simulink model "Dianlan_low_residence"  (R2021a)
settings: Solver=VariableStepAuto  StartTime=0.0  StopTime=20e-6  RelTol=1e-3
libraries: spsGroundLib x4, spsSeriesRLCBranchLib x3, spsVoltageMeasurementLib x3, spsDistributedParametersLineLib x2, spsControlledVoltageSourceLib x1, spspowerguiLib x1
settings Model: Creator=张瑞  LastModifiedBy=张瑞

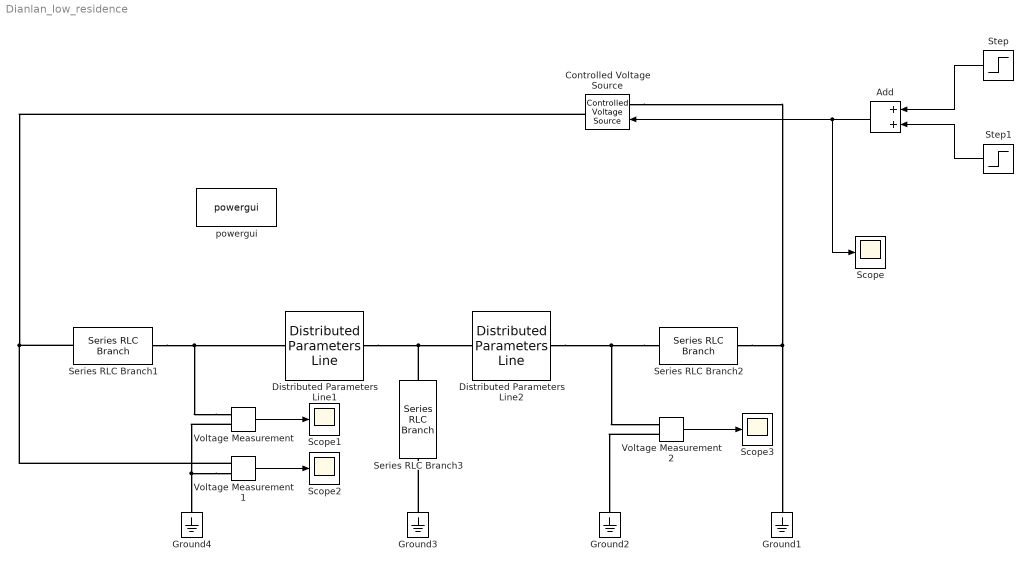
== system Dianlan_low_residence ==
  Add : Sum
  Controlled Voltage Source : spsControlledVoltageSourceLib/Controlled Voltage Source  Initialize=off  Source_Type=AC  Amplitude=0  Phase=0  Frequency=0  Measurements=Voltage
  Distributed Parameters Line1 : spsDistributedParametersLineLib/Distributed Parameters Line  Phases=1  Length=0.01  Frequency=1000  Resistance=1.8E-1  Inductance=2.75E-4  Capacitance=5.57E-7  x1=[-1.3e-07 0;-1.2e-07 0;-1.1e-07 0;-1e-07 0;-9e-08 0;-8e-08 0;-7e-08 0;-6e-08 0;-5e-08 0;-4e-08 0;-3e-08 0;-2e-08 0;-1e-08 0]  x2=[-1.3e-07 0;-1.2e-07 0;-1.1e-07 0;-1e-07 0;-9e-08 0;-8e-08 0;-7e-08 0;-6e-08 0;-5e-08 0;-4e-08 0;-3e-08 0;-2e-08 0;-1e-08 0]  x3=[-1.3e-07 0;-1.2e-07 0;-1.1e-07 0;-1e-07 0;-9e-08 0;-8e-08 0;-7e-08 0;-6e-08 0;-5e-08 0;-4e-08 0;-3e-08 0;-2e-08 0;-1e-08 0]  x4=[-1.3e-07 0;-1.2e-07 0;-1.1e-07 0;-1e-07 0;-9e-08 0;-8e-08 0;-7e-08 0;-6e-08 0;-5e-08 0;-4e-08 0;-3e-08 0;-2e-08 0;-1e-08 0]  x5=1.23763888109577e-07  V1=ones(3,3)  V2=ones(3,3)  I1=ones(3,3)  I2=ones(3,3)  nHarmo=1  Measurements=Phase-to-ground voltages  Decoupling=off  VsMag0=0  VrMag0=0  VsAngle0=0  VrAngle0=0  IsMag0=0  IrMag0=0  IsAngle0=0  IrAngle0=0
      settings: SourceProductBaseCode=PS
  Distributed Parameters Line2 : spsDistributedParametersLineLib/Distributed Parameters Line  Phases=1  Length=1.99  Frequency=1000  Resistance=1.8E-1  Inductance=2.75E-4  Capacitance=5.57E-7  x1=[-2.463e-05 0;-2.462e-05 0;-2.461e-05 0;-2.46e-05 0;-2.459e-05 0;-2.458e-05 0;-2.457e-05 0;-2.456e-05 0;-2.455e-05 0;-2.454e-05 0;-2.453e-05 0;-2.452e-05 0;-2.451e-05 0;-2.45e-05 0;-2.449e-05 0;-2.448e-05 0;-2.447e-05 0;-2.446e-05 0;-2.445e-05 0;-2.444e-05 0;-2.443e-05 0;-2.442e-05 0;-2.441e-05 0;-2.44e-05 0;-2.439e-05 0;-2.438e-05 0;-2.437e-05 0;-2.436e-05 0;-2.435e-05 0;-2.434e-05 0;-2.433e-05 0;-2.432e-05 0;-2.431e-05 0;-2.43e-05 0;-2.429e-05 0;-2.428e-05 0;-2.427e-05 0;-2.426e-05 0;-2.425e-05 0;-2.424e-05 0;-2.423e-05 0;-2.422e-05 0;-2.421e-05 0;-2.42e-05 0;-2.419e-05 0;-2.418e-05 0;-2.417e-05 0;-2.416e-05 0;-2.415e-05 0;-2.414e-05 0;-2.413e-05 0;-2.412e-05 0;-2.411e-05 0;-2.41e-05 0;-2.409e-05 0;-2.408e-05 0;-2.407e-05 0;-2.406e-05 0;-2.405e-05 0;-2.404e-05 0;-2.403e-05 0;-2.402e-05 0;-2.401e-05 0;-2.4e-05 0;-2.399e-05 0;-2.398e-05 0;-2.397e-05 0;-2.396e-05 0;-2.395e-05 0;-2.394e-05 0;-2.393e-05 0;-2.392e-05 0;-2.391e-05 0;-2.39e-05 0;-2.389e-05 0;-2.388e-05 0;-2.387e-05 0;-2.386e-05 0;-2.385e-05 0;-2.384e-05 0;-2.383e-05 0;-2.382e-05 0;-2.381e-05 0;-2.38e-05 0;-2.379e-05 0;-2.378e-05 0;-2.377e-05 0;-2.376e-05 0;-2.375e-05 0;-2.374e-05 0;-2.373e-05 0;-2.372e-05 0;-2.371e-05 0;-2.37e-05 0;-2.369e-05 0;-2.368e-05 0;-2.367e-05 0;-2.366e-05 0;-2.365e-05 0;-2.364e-05 0;-2.363e-05 0;-2.362e-05 0;-2.361e-05 0;-2.36e-05 0;-2.359e-05 0;-2.358e-05 0;-2.357e-05 0;-2.356e-05 0;-2.355e-05 0;-2.354e-05 0;-2.353e-05 0;-2.352e-05 0;-2.351e-05 0;-2.35e-05 0;-2.349e-05 0;-2.348e-05 0;-2.347e-05 0;-2.346e-05 0;-2.345e-05 0;-2.344e-05 0;-2.343e-05 0;-2.342e-05 0;-2.341e-05 0;-2.34e-05 0;-2.339e-05 0;-2.338e-05 0;-2.337e-05 0;-2.336e-05 0;-2.335e-05 0;-2.334e-05 0;-2.333e-05 0;-2.332e-05 0;-2.331e-05 0;-2.33e-05 0;-2.329e-05 0;-2.328e-05 0;-2.327e-05 0;-2.326e-05 0;-2.325e-05 0;-2.324e-05 0;-2.323e-05 0;-2.322e-05 0;-2.321e-05 0;-2.32e-05 0;-2.319e-05 0;-2.318e-05 0;-2.317e-05 0;-2.316e-05 0;-2.315e-05 0;-2.314e-05 0;-2.313e-05 0;-2.312e-05 0;-2.311e-05 0;-2.31e-05 0;-2.309e-05 0;-2.308e-05 0;-2.307e-05 0;-2.306e-05 0;-2.305e-05 0;-2.304e-05 0;-2.303e-05 0;-2.302e-05 0;-2.301e-05 0;-2.3e-05 0;-2.299e-05 0;-2.298e-05 0;-2.297e-05 0;-2.296e-05 0;-2.295e-05 0;-2.294e-05 0;-2.293e-05 0;-2.292e-05 0;-2.291e-05 0;-2.29e-05 0;-2.289e-05 0;-2.288e-05 0;-2.287e-05 0;-2.286e-05 0;-2.285e-05 0;-2.284e-05 0;-2.283e-05 0;-2.282e-05 0;-2.281e-05 0;-2.28e-05 0;-2.279e-05 0;-2.278e-05 0;-2.277e-05 0;-2.276e-05 0;-2.275e-05 0;-2.274e-05 0;-2.273e-05 0;-2.272e-05 0;-2.271e-05 0;-2.27e-05 0;-2.269e-05 0;-2.268e-05 0;-2.267e-05 0;-2.266e-05 0;-2.265e-05 0;-2.264e-05 0;-2.263e-05 0;-2.262e-05 0;-2.261e-05 0;-2.26e-05 0;-2.259e-05 0;-2.258e-05 0;-2.257e-05 0;-2.256e-05 0;-2.255e-05 0;-2.254e-05 0;-2.253e-05 0;-2.252e-05 0;-2.251e-05 0;-2.25e-05 0;-2.249e-05 0;-2.248e-05 0;-2.247e-05 0;-2.246e-05 0;-2.245e-05 0;-2.244e-05 0;-2.243e-05 0;-2.242e-05 0;-2.241e-05 0;-2.24e-05 0;-2.239e-05 0;-2.238e-05 0;-2.237e-05 0;-2.236e-05 0;-2.235e-05 0;-2.234e-05 0;-2.233e-05 0;-2.232e-05 0;-2.231e-05 0;-2.23e-05 0;-2.229e-05 0;-2.228e-05 0;-2.227e-05 0;-2.226e-05 0;-2.225e-05 0;-2.224e-05 0;-2.223e-05 0;-2.222e-05 0;-2.221e-05 0;-2.22e-05 0;-2.219e-05 0;-2.218e-05 0;-2.217e-05 0;-2.216e-05 0;-2.215e-05 0;-2.214e-05 0;-2.213e-05 0;-2.212e-05 0;-2.211e-05 0;-2.21e-05 0;-2.209e-05 0;-2.208e-05 0;-2.207e-05 0;-2.206e-05 0;-2.205e-05 0;-2.204e-05 0;-2.203e-05 0;-2.202e-05 0;-2.201e-05 0;-2.2e-05 0;-2.199e-05 0;-2.198e-05 0;-2.197e-05 0;-2.196e-05 0;-2.195e-05 0;-2.194e-05 0;-2.193e-05 0;-2.192e-05 0;-2.191e-05 0;-2.19e-05 0;-2.189e-05 0;-2.188e-05 0;-2.187e-05 0;-2.186e-05 0;-2.185e-05 0;-2.184e-05 0;-2.183e-05 0;-2.182e-05 0;-2.181e-05 0;-2.18e-05 0;-2.179e-05 0;-2.178e-05 0;-2.177e-05 0;-2.176e-05 0;-2.175e-05 0;-2.174e-05 0;-2.173e-05 0;-2.172e-05 0;-2.171e-05 0;-2.17e-05 0;-2.169e-05 0;-2.168e-05 0;-2.167e-05 0;-2.166e-05 0;-2.165e-05 0;-2.164e-05 0;-2.163e-05 0;-2.162e-05 0;-2.161e-05 0;-2.16e-05 0;-2.159e-05 0;-2.158e-05 0;-2.157e-05 0;-2.156e-05 0;-2.155e-05 0;-2.154e-05 0 ...(+26615 chars)]  x2=[-2.463e-05 0;-2.462e-05 0;-2.461e-05 0;-2.46e-05 0;-2.459e-05 0;-2.458e-05 0;-2.457e-05 0;-2.456e-05 0;-2.455e-05 0;-2.454e-05 0;-2.453e-05 0;-2.452e-05 0;-2.451e-05 0;-2.45e-05 0;-2.449e-05 0;-2.448e-05 0;-2.447e-05 0;-2.446e-05 0;-2.445e-05 0;-2.444e-05 0;-2.443e-05 0;-2.442e-05 0;-2.441e-05 0;-2.44e-05 0;-2.439e-05 0;-2.438e-05 0;-2.437e-05 0;-2.436e-05 0;-2.435e-05 0;-2.434e-05 0;-2.433e-05 0;-2.432e-05 0;-2.431e-05 0;-2.43e-05 0;-2.429e-05 0;-2.428e-05 0;-2.427e-05 0;-2.426e-05 0;-2.425e-05 0;-2.424e-05 0;-2.423e-05 0;-2.422e-05 0;-2.421e-05 0;-2.42e-05 0;-2.419e-05 0;-2.418e-05 0;-2.417e-05 0;-2.416e-05 0;-2.415e-05 0;-2.414e-05 0;-2.413e-05 0;-2.412e-05 0;-2.411e-05 0;-2.41e-05 0;-2.409e-05 0;-2.408e-05 0;-2.407e-05 0;-2.406e-05 0;-2.405e-05 0;-2.404e-05 0;-2.403e-05 0;-2.402e-05 0;-2.401e-05 0;-2.4e-05 0;-2.399e-05 0;-2.398e-05 0;-2.397e-05 0;-2.396e-05 0;-2.395e-05 0;-2.394e-05 0;-2.393e-05 0;-2.392e-05 0;-2.391e-05 0;-2.39e-05 0;-2.389e-05 0;-2.388e-05 0;-2.387e-05 0;-2.386e-05 0;-2.385e-05 0;-2.384e-05 0;-2.383e-05 0;-2.382e-05 0;-2.381e-05 0;-2.38e-05 0;-2.379e-05 0;-2.378e-05 0;-2.377e-05 0;-2.376e-05 0;-2.375e-05 0;-2.374e-05 0;-2.373e-05 0;-2.372e-05 0;-2.371e-05 0;-2.37e-05 0;-2.369e-05 0;-2.368e-05 0;-2.367e-05 0;-2.366e-05 0;-2.365e-05 0;-2.364e-05 0;-2.363e-05 0;-2.362e-05 0;-2.361e-05 0;-2.36e-05 0;-2.359e-05 0;-2.358e-05 0;-2.357e-05 0;-2.356e-05 0;-2.355e-05 0;-2.354e-05 0;-2.353e-05 0;-2.352e-05 0;-2.351e-05 0;-2.35e-05 0;-2.349e-05 0;-2.348e-05 0;-2.347e-05 0;-2.346e-05 0;-2.345e-05 0;-2.344e-05 0;-2.343e-05 0;-2.342e-05 0;-2.341e-05 0;-2.34e-05 0;-2.339e-05 0;-2.338e-05 0;-2.337e-05 0;-2.336e-05 0;-2.335e-05 0;-2.334e-05 0;-2.333e-05 0;-2.332e-05 0;-2.331e-05 0;-2.33e-05 0;-2.329e-05 0;-2.328e-05 0;-2.327e-05 0;-2.326e-05 0;-2.325e-05 0;-2.324e-05 0;-2.323e-05 0;-2.322e-05 0;-2.321e-05 0;-2.32e-05 0;-2.319e-05 0;-2.318e-05 0;-2.317e-05 0;-2.316e-05 0;-2.315e-05 0;-2.314e-05 0;-2.313e-05 0;-2.312e-05 0;-2.311e-05 0;-2.31e-05 0;-2.309e-05 0;-2.308e-05 0;-2.307e-05 0;-2.306e-05 0;-2.305e-05 0;-2.304e-05 0;-2.303e-05 0;-2.302e-05 0;-2.301e-05 0;-2.3e-05 0;-2.299e-05 0;-2.298e-05 0;-2.297e-05 0;-2.296e-05 0;-2.295e-05 0;-2.294e-05 0;-2.293e-05 0;-2.292e-05 0;-2.291e-05 0;-2.29e-05 0;-2.289e-05 0;-2.288e-05 0;-2.287e-05 0;-2.286e-05 0;-2.285e-05 0;-2.284e-05 0;-2.283e-05 0;-2.282e-05 0;-2.281e-05 0;-2.28e-05 0;-2.279e-05 0;-2.278e-05 0;-2.277e-05 0;-2.276e-05 0;-2.275e-05 0;-2.274e-05 0;-2.273e-05 0;-2.272e-05 0;-2.271e-05 0;-2.27e-05 0;-2.269e-05 0;-2.268e-05 0;-2.267e-05 0;-2.266e-05 0;-2.265e-05 0;-2.264e-05 0;-2.263e-05 0;-2.262e-05 0;-2.261e-05 0;-2.26e-05 0;-2.259e-05 0;-2.258e-05 0;-2.257e-05 0;-2.256e-05 0;-2.255e-05 0;-2.254e-05 0;-2.253e-05 0;-2.252e-05 0;-2.251e-05 0;-2.25e-05 0;-2.249e-05 0;-2.248e-05 0;-2.247e-05 0;-2.246e-05 0;-2.245e-05 0;-2.244e-05 0;-2.243e-05 0;-2.242e-05 0;-2.241e-05 0;-2.24e-05 0;-2.239e-05 0;-2.238e-05 0;-2.237e-05 0;-2.236e-05 0;-2.235e-05 0;-2.234e-05 0;-2.233e-05 0;-2.232e-05 0;-2.231e-05 0;-2.23e-05 0;-2.229e-05 0;-2.228e-05 0;-2.227e-05 0;-2.226e-05 0;-2.225e-05 0;-2.224e-05 0;-2.223e-05 0;-2.222e-05 0;-2.221e-05 0;-2.22e-05 0;-2.219e-05 0;-2.218e-05 0;-2.217e-05 0;-2.216e-05 0;-2.215e-05 0;-2.214e-05 0;-2.213e-05 0;-2.212e-05 0;-2.211e-05 0;-2.21e-05 0;-2.209e-05 0;-2.208e-05 0;-2.207e-05 0;-2.206e-05 0;-2.205e-05 0;-2.204e-05 0;-2.203e-05 0;-2.202e-05 0;-2.201e-05 0;-2.2e-05 0;-2.199e-05 0;-2.198e-05 0;-2.197e-05 0;-2.196e-05 0;-2.195e-05 0;-2.194e-05 0;-2.193e-05 0;-2.192e-05 0;-2.191e-05 0;-2.19e-05 0;-2.189e-05 0;-2.188e-05 0;-2.187e-05 0;-2.186e-05 0;-2.185e-05 0;-2.184e-05 0;-2.183e-05 0;-2.182e-05 0;-2.181e-05 0;-2.18e-05 0;-2.179e-05 0;-2.178e-05 0;-2.177e-05 0;-2.176e-05 0;-2.175e-05 0;-2.174e-05 0;-2.173e-05 0;-2.172e-05 0;-2.171e-05 0;-2.17e-05 0;-2.169e-05 0;-2.168e-05 0;-2.167e-05 0;-2.166e-05 0;-2.165e-05 0;-2.164e-05 0;-2.163e-05 0;-2.162e-05 0;-2.161e-05 0;-2.16e-05 0;-2.159e-05 0;-2.158e-05 0;-2.157e-05 0;-2.156e-05 0;-2.155e-05 0;-2.154e-05 0 ...(+26615 chars)]  x3=[-2.463e-05 0;-2.462e-05 0;-2.461e-05 0;-2.46e-05 0;-2.459e-05 0;-2.458e-05 0;-2.457e-05 0;-2.456e-05 0;-2.455e-05 0;-2.454e-05 0;-2.453e-05 0;-2.452e-05 0;-2.451e-05 0;-2.45e-05 0;-2.449e-05 0;-2.448e-05 0;-2.447e-05 0;-2.446e-05 0;-2.445e-05 0;-2.444e-05 0;-2.443e-05 0;-2.442e-05 0;-2.441e-05 0;-2.44e-05 0;-2.439e-05 0;-2.438e-05 0;-2.437e-05 0;-2.436e-05 0;-2.435e-05 0;-2.434e-05 0;-2.433e-05 0;-2.432e-05 0;-2.431e-05 0;-2.43e-05 0;-2.429e-05 0;-2.428e-05 0;-2.427e-05 0;-2.426e-05 0;-2.425e-05 0;-2.424e-05 0;-2.423e-05 0;-2.422e-05 0;-2.421e-05 0;-2.42e-05 0;-2.419e-05 0;-2.418e-05 0;-2.417e-05 0;-2.416e-05 0;-2.415e-05 0;-2.414e-05 0;-2.413e-05 0;-2.412e-05 0;-2.411e-05 0;-2.41e-05 0;-2.409e-05 0;-2.408e-05 0;-2.407e-05 0;-2.406e-05 0;-2.405e-05 0;-2.404e-05 0;-2.403e-05 0;-2.402e-05 0;-2.401e-05 0;-2.4e-05 0;-2.399e-05 0;-2.398e-05 0;-2.397e-05 0;-2.396e-05 0;-2.395e-05 0;-2.394e-05 0;-2.393e-05 0;-2.392e-05 0;-2.391e-05 0;-2.39e-05 0;-2.389e-05 0;-2.388e-05 0;-2.387e-05 0;-2.386e-05 0;-2.385e-05 0;-2.384e-05 0;-2.383e-05 0;-2.382e-05 0;-2.381e-05 0;-2.38e-05 0;-2.379e-05 0;-2.378e-05 0;-2.377e-05 0;-2.376e-05 0;-2.375e-05 0;-2.374e-05 0;-2.373e-05 0;-2.372e-05 0;-2.371e-05 0;-2.37e-05 0;-2.369e-05 0;-2.368e-05 0;-2.367e-05 0;-2.366e-05 0;-2.365e-05 0;-2.364e-05 0;-2.363e-05 0;-2.362e-05 0;-2.361e-05 0;-2.36e-05 0;-2.359e-05 0;-2.358e-05 0;-2.357e-05 0;-2.356e-05 0;-2.355e-05 0;-2.354e-05 0;-2.353e-05 0;-2.352e-05 0;-2.351e-05 0;-2.35e-05 0;-2.349e-05 0;-2.348e-05 0;-2.347e-05 0;-2.346e-05 0;-2.345e-05 0;-2.344e-05 0;-2.343e-05 0;-2.342e-05 0;-2.341e-05 0;-2.34e-05 0;-2.339e-05 0;-2.338e-05 0;-2.337e-05 0;-2.336e-05 0;-2.335e-05 0;-2.334e-05 0;-2.333e-05 0;-2.332e-05 0;-2.331e-05 0;-2.33e-05 0;-2.329e-05 0;-2.328e-05 0;-2.327e-05 0;-2.326e-05 0;-2.325e-05 0;-2.324e-05 0;-2.323e-05 0;-2.322e-05 0;-2.321e-05 0;-2.32e-05 0;-2.319e-05 0;-2.318e-05 0;-2.317e-05 0;-2.316e-05 0;-2.315e-05 0;-2.314e-05 0;-2.313e-05 0;-2.312e-05 0;-2.311e-05 0;-2.31e-05 0;-2.309e-05 0;-2.308e-05 0;-2.307e-05 0;-2.306e-05 0;-2.305e-05 0;-2.304e-05 0;-2.303e-05 0;-2.302e-05 0;-2.301e-05 0;-2.3e-05 0;-2.299e-05 0;-2.298e-05 0;-2.297e-05 0;-2.296e-05 0;-2.295e-05 0;-2.294e-05 0;-2.293e-05 0;-2.292e-05 0;-2.291e-05 0;-2.29e-05 0;-2.289e-05 0;-2.288e-05 0;-2.287e-05 0;-2.286e-05 0;-2.285e-05 0;-2.284e-05 0;-2.283e-05 0;-2.282e-05 0;-2.281e-05 0;-2.28e-05 0;-2.279e-05 0;-2.278e-05 0;-2.277e-05 0;-2.276e-05 0;-2.275e-05 0;-2.274e-05 0;-2.273e-05 0;-2.272e-05 0;-2.271e-05 0;-2.27e-05 0;-2.269e-05 0;-2.268e-05 0;-2.267e-05 0;-2.266e-05 0;-2.265e-05 0;-2.264e-05 0;-2.263e-05 0;-2.262e-05 0;-2.261e-05 0;-2.26e-05 0;-2.259e-05 0;-2.258e-05 0;-2.257e-05 0;-2.256e-05 0;-2.255e-05 0;-2.254e-05 0;-2.253e-05 0;-2.252e-05 0;-2.251e-05 0;-2.25e-05 0;-2.249e-05 0;-2.248e-05 0;-2.247e-05 0;-2.246e-05 0;-2.245e-05 0;-2.244e-05 0;-2.243e-05 0;-2.242e-05 0;-2.241e-05 0;-2.24e-05 0;-2.239e-05 0;-2.238e-05 0;-2.237e-05 0;-2.236e-05 0;-2.235e-05 0;-2.234e-05 0;-2.233e-05 0;-2.232e-05 0;-2.231e-05 0;-2.23e-05 0;-2.229e-05 0;-2.228e-05 0;-2.227e-05 0;-2.226e-05 0;-2.225e-05 0;-2.224e-05 0;-2.223e-05 0;-2.222e-05 0;-2.221e-05 0;-2.22e-05 0;-2.219e-05 0;-2.218e-05 0;-2.217e-05 0;-2.216e-05 0;-2.215e-05 0;-2.214e-05 0;-2.213e-05 0;-2.212e-05 0;-2.211e-05 0;-2.21e-05 0;-2.209e-05 0;-2.208e-05 0;-2.207e-05 0;-2.206e-05 0;-2.205e-05 0;-2.204e-05 0;-2.203e-05 0;-2.202e-05 0;-2.201e-05 0;-2.2e-05 0;-2.199e-05 0;-2.198e-05 0;-2.197e-05 0;-2.196e-05 0;-2.195e-05 0;-2.194e-05 0;-2.193e-05 0;-2.192e-05 0;-2.191e-05 0;-2.19e-05 0;-2.189e-05 0;-2.188e-05 0;-2.187e-05 0;-2.186e-05 0;-2.185e-05 0;-2.184e-05 0;-2.183e-05 0;-2.182e-05 0;-2.181e-05 0;-2.18e-05 0;-2.179e-05 0;-2.178e-05 0;-2.177e-05 0;-2.176e-05 0;-2.175e-05 0;-2.174e-05 0;-2.173e-05 0;-2.172e-05 0;-2.171e-05 0;-2.17e-05 0;-2.169e-05 0;-2.168e-05 0;-2.167e-05 0;-2.166e-05 0;-2.165e-05 0;-2.164e-05 0;-2.163e-05 0;-2.162e-05 0;-2.161e-05 0;-2.16e-05 0;-2.159e-05 0;-2.158e-05 0;-2.157e-05 0;-2.156e-05 0;-2.155e-05 0;-2.154e-05 0 ...(+26615 chars)]  x4=[-2.463e-05 0;-2.462e-05 0;-2.461e-05 0;-2.46e-05 0;-2.459e-05 0;-2.458e-05 0;-2.457e-05 0;-2.456e-05 0;-2.455e-05 0;-2.454e-05 0;-2.453e-05 0;-2.452e-05 0;-2.451e-05 0;-2.45e-05 0;-2.449e-05 0;-2.448e-05 0;-2.447e-05 0;-2.446e-05 0;-2.445e-05 0;-2.444e-05 0;-2.443e-05 0;-2.442e-05 0;-2.441e-05 0;-2.44e-05 0;-2.439e-05 0;-2.438e-05 0;-2.437e-05 0;-2.436e-05 0;-2.435e-05 0;-2.434e-05 0;-2.433e-05 0;-2.432e-05 0;-2.431e-05 0;-2.43e-05 0;-2.429e-05 0;-2.428e-05 0;-2.427e-05 0;-2.426e-05 0;-2.425e-05 0;-2.424e-05 0;-2.423e-05 0;-2.422e-05 0;-2.421e-05 0;-2.42e-05 0;-2.419e-05 0;-2.418e-05 0;-2.417e-05 0;-2.416e-05 0;-2.415e-05 0;-2.414e-05 0;-2.413e-05 0;-2.412e-05 0;-2.411e-05 0;-2.41e-05 0;-2.409e-05 0;-2.408e-05 0;-2.407e-05 0;-2.406e-05 0;-2.405e-05 0;-2.404e-05 0;-2.403e-05 0;-2.402e-05 0;-2.401e-05 0;-2.4e-05 0;-2.399e-05 0;-2.398e-05 0;-2.397e-05 0;-2.396e-05 0;-2.395e-05 0;-2.394e-05 0;-2.393e-05 0;-2.392e-05 0;-2.391e-05 0;-2.39e-05 0;-2.389e-05 0;-2.388e-05 0;-2.387e-05 0;-2.386e-05 0;-2.385e-05 0;-2.384e-05 0;-2.383e-05 0;-2.382e-05 0;-2.381e-05 0;-2.38e-05 0;-2.379e-05 0;-2.378e-05 0;-2.377e-05 0;-2.376e-05 0;-2.375e-05 0;-2.374e-05 0;-2.373e-05 0;-2.372e-05 0;-2.371e-05 0;-2.37e-05 0;-2.369e-05 0;-2.368e-05 0;-2.367e-05 0;-2.366e-05 0;-2.365e-05 0;-2.364e-05 0;-2.363e-05 0;-2.362e-05 0;-2.361e-05 0;-2.36e-05 0;-2.359e-05 0;-2.358e-05 0;-2.357e-05 0;-2.356e-05 0;-2.355e-05 0;-2.354e-05 0;-2.353e-05 0;-2.352e-05 0;-2.351e-05 0;-2.35e-05 0;-2.349e-05 0;-2.348e-05 0;-2.347e-05 0;-2.346e-05 0;-2.345e-05 0;-2.344e-05 0;-2.343e-05 0;-2.342e-05 0;-2.341e-05 0;-2.34e-05 0;-2.339e-05 0;-2.338e-05 0;-2.337e-05 0;-2.336e-05 0;-2.335e-05 0;-2.334e-05 0;-2.333e-05 0;-2.332e-05 0;-2.331e-05 0;-2.33e-05 0;-2.329e-05 0;-2.328e-05 0;-2.327e-05 0;-2.326e-05 0;-2.325e-05 0;-2.324e-05 0;-2.323e-05 0;-2.322e-05 0;-2.321e-05 0;-2.32e-05 0;-2.319e-05 0;-2.318e-05 0;-2.317e-05 0;-2.316e-05 0;-2.315e-05 0;-2.314e-05 0;-2.313e-05 0;-2.312e-05 0;-2.311e-05 0;-2.31e-05 0;-2.309e-05 0;-2.308e-05 0;-2.307e-05 0;-2.306e-05 0;-2.305e-05 0;-2.304e-05 0;-2.303e-05 0;-2.302e-05 0;-2.301e-05 0;-2.3e-05 0;-2.299e-05 0;-2.298e-05 0;-2.297e-05 0;-2.296e-05 0;-2.295e-05 0;-2.294e-05 0;-2.293e-05 0;-2.292e-05 0;-2.291e-05 0;-2.29e-05 0;-2.289e-05 0;-2.288e-05 0;-2.287e-05 0;-2.286e-05 0;-2.285e-05 0;-2.284e-05 0;-2.283e-05 0;-2.282e-05 0;-2.281e-05 0;-2.28e-05 0;-2.279e-05 0;-2.278e-05 0;-2.277e-05 0;-2.276e-05 0;-2.275e-05 0;-2.274e-05 0;-2.273e-05 0;-2.272e-05 0;-2.271e-05 0;-2.27e-05 0;-2.269e-05 0;-2.268e-05 0;-2.267e-05 0;-2.266e-05 0;-2.265e-05 0;-2.264e-05 0;-2.263e-05 0;-2.262e-05 0;-2.261e-05 0;-2.26e-05 0;-2.259e-05 0;-2.258e-05 0;-2.257e-05 0;-2.256e-05 0;-2.255e-05 0;-2.254e-05 0;-2.253e-05 0;-2.252e-05 0;-2.251e-05 0;-2.25e-05 0;-2.249e-05 0;-2.248e-05 0;-2.247e-05 0;-2.246e-05 0;-2.245e-05 0;-2.244e-05 0;-2.243e-05 0;-2.242e-05 0;-2.241e-05 0;-2.24e-05 0;-2.239e-05 0;-2.238e-05 0;-2.237e-05 0;-2.236e-05 0;-2.235e-05 0;-2.234e-05 0;-2.233e-05 0;-2.232e-05 0;-2.231e-05 0;-2.23e-05 0;-2.229e-05 0;-2.228e-05 0;-2.227e-05 0;-2.226e-05 0;-2.225e-05 0;-2.224e-05 0;-2.223e-05 0;-2.222e-05 0;-2.221e-05 0;-2.22e-05 0;-2.219e-05 0;-2.218e-05 0;-2.217e-05 0;-2.216e-05 0;-2.215e-05 0;-2.214e-05 0;-2.213e-05 0;-2.212e-05 0;-2.211e-05 0;-2.21e-05 0;-2.209e-05 0;-2.208e-05 0;-2.207e-05 0;-2.206e-05 0;-2.205e-05 0;-2.204e-05 0;-2.203e-05 0;-2.202e-05 0;-2.201e-05 0;-2.2e-05 0;-2.199e-05 0;-2.198e-05 0;-2.197e-05 0;-2.196e-05 0;-2.195e-05 0;-2.194e-05 0;-2.193e-05 0;-2.192e-05 0;-2.191e-05 0;-2.19e-05 0;-2.189e-05 0;-2.188e-05 0;-2.187e-05 0;-2.186e-05 0;-2.185e-05 0;-2.184e-05 0;-2.183e-05 0;-2.182e-05 0;-2.181e-05 0;-2.18e-05 0;-2.179e-05 0;-2.178e-05 0;-2.177e-05 0;-2.176e-05 0;-2.175e-05 0;-2.174e-05 0;-2.173e-05 0;-2.172e-05 0;-2.171e-05 0;-2.17e-05 0;-2.169e-05 0;-2.168e-05 0;-2.167e-05 0;-2.166e-05 0;-2.165e-05 0;-2.164e-05 0;-2.163e-05 0;-2.162e-05 0;-2.161e-05 0;-2.16e-05 0;-2.159e-05 0;-2.158e-05 0;-2.157e-05 0;-2.156e-05 0;-2.155e-05 0;-2.154e-05 0 ...(+26615 chars)]  x5=2.46290137338059e-05  V1=ones(3,3)  V2=ones(3,3)  I1=ones(3,3)  I2=ones(3,3)  nHarmo=1  Measurements=Phase-to-ground voltages  Decoupling=off  VsMag0=0  VrMag0=0  VsAngle0=0  VrAngle0=0  IsMag0=0  IrMag0=0  IsAngle0=0  IrAngle0=0
      settings: SourceProductBaseCode=PS
  Ground{1..4} (4 alike) : spsGroundLib/Ground  LConnTagsString=a
  Scope{,1..3} (4 alike) : Scope
  Series RLC Branch1 : spsSeriesRLCBranchLib/Series RLC Branch  LConnTagsString=__new0  RConnTagsString=__new0  BranchType=R  Resistance=1  Inductance=1e-3  SetiL0=off  InitialCurrent=0  Capacitance=1e-6  Setx0=off  InitialVoltage=0  Measurements=None
  Series RLC Branch2 : spsSeriesRLCBranchLib/Series RLC Branch  LConnTagsString=__new0  RConnTagsString=__new0  BranchType=R  Resistance=22.2  Inductance=1e-3  SetiL0=off  InitialCurrent=0  Capacitance=1e-6  Setx0=off  InitialVoltage=0  Measurements=None
  Series RLC Branch3 : spsSeriesRLCBranchLib/Series RLC Branch  LConnTagsString=__new0  RConnTagsString=__new0  BranchType=R  Resistance=0.001  Inductance=1e-3  SetiL0=off  InitialCurrent=0  Capacitance=1e-6  Setx0=off  InitialVoltage=0  Measurements=None
  Step : Step  Time=0.3E-6  Before=28  After=0  SampleTime=1E-08
  Step1 : Step  Time=0.1E-6  Before=-28  After=0  SampleTime=1E-08
  Voltage Measurement : spsVoltageMeasurementLib/Voltage Measurement  PhasorSimulation=off  OutputType=Complex  PSBequivalent=0
  Voltage Measurement1 : spsVoltageMeasurementLib/Voltage Measurement  PhasorSimulation=off  OutputType=Complex  PSBequivalent=0
  Voltage Measurement2 : spsVoltageMeasurementLib/Voltage Measurement  PhasorSimulation=off  OutputType=Complex  PSBequivalent=0
  powergui : spspowerguiLib/powergui  Priority=1  SimulationMode=Discrete  SampleTime=0.01e-6  frequency=60  Iterations=50  frequencyindice=0  Pbase=100e6  ErrMax=1e-4  UnitsV=kV  UnitsW=MW  buscounter=0  FunctionMessages=off  echomessages=off  EnableUseOfTLC=off  CurrentSourceSwitches=off  DisableSnubberDevices=off  DisableRonSwitches=off  DisableVfSwitches=off  DisplayEquations=off  AutomaticDiscreteSolvers=off  SolverType=Tustin/Backward Euler (TBE)  Interpol=off  ExternalGateDelay=off  methode=off  Ts=100  x0status=blocks  SPID=on  SwTol=0  HookPort=off  NonlinearTolerance=1e-4  nMaxIteration=100  ContinueOnMaxIteration=off  RestoreLinks=warning  ResistiveCurrentMeasurement=off  Frange=[0:2:500]  Ylog=off  Xlog=on  ShowGrid=off  save=off  variable=ZData  structure=0  ZoomFFT=off  StartTime=0.0  cycles=1  DisplayStyle=1  fundamental=60  FreqAxis=off  MaxFrequency=1000  frequencyindicesteady=1  RmsSteady=1  display=off
  wires:
  Voltage Measurement2/1 -> Scope3/1
  Voltage Measurement/1 -> Scope1/1
  Voltage Measurement1/1 -> Scope2/1
  Step1/1 -> Add/2
  Step/1 -> Add/1
  Add/1 -> Scope/1, Controlled Voltage Source/1
  connections:
  Voltage Measurement/LConn1 -- Distributed Parameters Line1/LConn1 -- Series RLC Branch1/RConn1
  Series RLC Branch1/LConn1 -- Controlled Voltage Source/RConn1 -- Voltage Measurement1/LConn1
  Controlled Voltage Source/LConn1 -- Series RLC Branch2/RConn1 -- Ground1/LConn1
  Series RLC Branch2/LConn1 -- Distributed Parameters Line2/RConn1 -- Voltage Measurement2/LConn1
  Distributed Parameters Line1/RConn1 -- Distributed Parameters Line2/LConn1 -- Series RLC Branch3/LConn1
  Voltage Measurement1/LConn2 -- Ground4/LConn1 -- Voltage Measurement/LConn2
  Voltage Measurement2/LConn2 -- Ground2/LConn1
  Ground3/LConn1 -- Series RLC Branch3/RConn1
